simulink model "CIC_manual_test"  (R2016b)
settings: Solver=VariableStepAuto  StartTime=0.0  StopTime=2^16/Fadc  RelTol=1e-3  EnableMultiTasking=on
PreLoadFcn:
  | setup
values from neighbouring files (symbols this model uses):
  Fadc = 614.4e6    (= 614400000)    [setup.m]
libraries: xbsIndex_r4 x26, CryoDetLibCMB x1
settings Model: Creator=Mitch  LastModifiedBy=mdewart
settings OptimizationCC: LifeSpan=inf
settings DebuggingCC: SFUnexpectedBacktrackingDiag=warning  SFNoUnconditionalDefaultTransitionDiag=warning  SFExecutionAtInitializationDiag=none
settings GRTTargetCC: TargetLangStandard=C89/C90 (ANSI)  GeneratePreprocessorConditionals=Disable all
settings ConfigComp: CovMetricSettings=dw  CovHtmlReporting=on  CovSaveCumulativeToWorkspaceVar=on  CovSaveSingleToWorkspaceVar=on  CovExternalEMLEnable=off

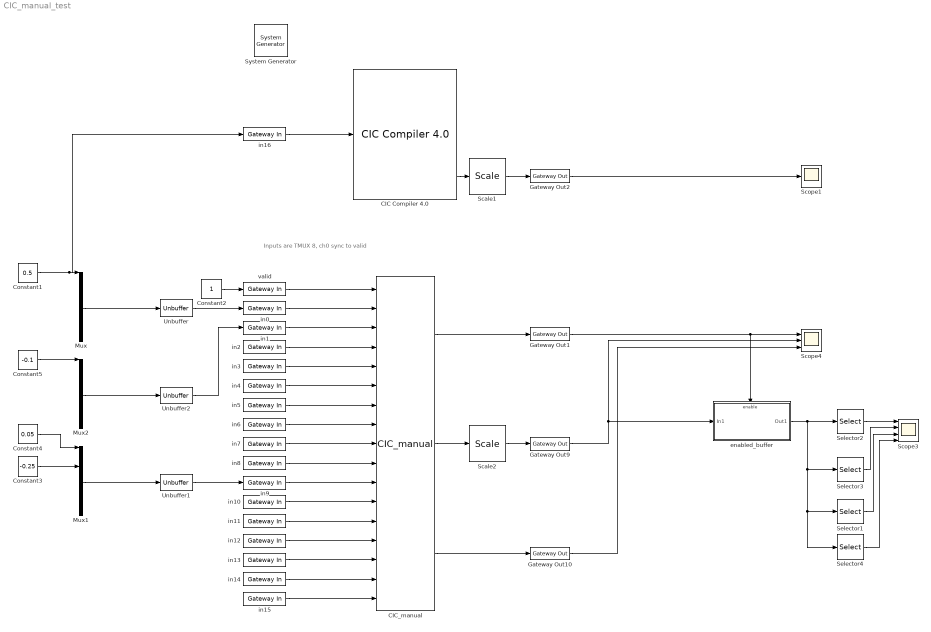
== system CIC_manual_test ==
  note: Inputs are TMUX 8, ch0 sync to valid
  " System Generator" : xbsIndex_r4/ System Generator  Tag=genX  xilinxfamily=kintexu  part=xcku040  speed=-2-e  package=ffva1156  synthesis_tool=Vivado  clock_wrapper=Clock Enables  directory=./netlist  proj_type=Vivado  Synth_file=Vivado Synthesis Defaults  Impl_file=Vivado Implementation Defaults  testbench=off  simulink_period=2/Fadc  sysclk_period=2e9/Fadc  dcm_input_clock_period=10  incr_netlist=off  trim_vbits=Everywhere in SubSystem  dbl_ovrd=According to Block Masks  core_generation=According to Block Masks  run_coregen=off  deprecated_control=off  eval_field=0  block_type=sysgen
  "CIC Compiler 4.0 " : xbsIndex_r4/CIC Compiler 4.0   filter_type=Decimation  number_of_stages=3  differential_delay=1  number_of_channels=1  sample_rate_changes=Fixed  fixed_or_initial_rate=16  minimum_rate=16  maximum_rate=16  ratespecification=Hardware_Oversampling_Rate  sampleperiod=1  hardwareoversamplingrate=1  quantization=Full_Precision  output_data_width=30  use_xtreme_dsp_slice=on  use_streaming_interface=on  has_aclken=off  has_aresetn=off  has_dout_tready=off  trim_axipin_name=on  gui_behaviour=Sysgen_GUI  input_data_width=18  ip_name=CIC Compiler  ip_version=4.0  dsptool_ready=true  wrapper_available=true  port_translation_map={ 'aclken' => 'en', 'aresetn' => 'rst' }  ipcore_xco_need_fpga_part=true  ipcore_verbose=false  block_type=cic_compiler_v4_0
  CIC_manual : CryoDetLibCMB/CIC_manual  n_bit=30  b_pt=15
  Constant1 : Constant  Value=0.5  SampleTime=16/Fadc
  Constant2 : Constant  SampleTime=2/Fadc
  Constant3 : Constant  Value=-0.25  SampleTime=16/Fadc
  Constant4 : Constant  Value=0.05  SampleTime=16/Fadc
  Constant5 : Constant  Value=-0.1  SampleTime=16/Fadc
  Gateway Out{1..2,9..10} (4 alike) : xbsIndex_r4/Gateway Out  inherit_from_input=off  hdl_port=on  rows=1  columns=1  UseAsDAC=off  DACChannel='1'  interface=None  automatic_assignment=on  address_offset=hex2dec('00')  intf_name=''  intf_description=''  timing_constraint=None  locs_specified=off  LOCs={}  io_standard={}  block_type=gatewayout
  Mux : Mux  Inputs=8
  Mux1 : Mux  Inputs=8
  Mux2 : Mux  Inputs=8
  Scale1 : xbsIndex_r4/Scale  scale_factor=-12  dbl_ovrd=off  block_type=scale
  Scale2 : xbsIndex_r4/Scale  scale_factor=-12  dbl_ovrd=off  block_type=scale
  Scope1 : Scope
  Scope3 : Scope  NumInputPorts=4
  Scope4 : Scope  NumInputPorts=3
  Selector1 : Selector  InputPortWidth=128  IndexOptions=Index vector (dialog)  Indices=[9+1]  OutputSizes=1
  Selector2 : Selector  InputPortWidth=128  IndexOptions=Index vector (dialog)  Indices=[0+1]  OutputSizes=1
  Selector3 : Selector  InputPortWidth=128  IndexOptions=Index vector (dialog)  Indices=[1+1]  OutputSizes=1
  Selector4 : Selector  InputPortWidth=128  IndexOptions=Index vector (dialog)  Indices=[41+1]  OutputSizes=1
  Unbuffer : Unbuffer  SampleBasedProcessing=Same as frame based
  Unbuffer1 : Unbuffer  SampleBasedProcessing=Same as frame based
  Unbuffer2 : Unbuffer  SampleBasedProcessing=Same as frame based
  enabled_buffer : Subsystem
  in{0..15} (16 alike) : xbsIndex_r4/Gateway In  gui_display_data_type=Fixed-point  arith_type="Signed  (2's comp)"  n_bits=18  bin_pt=15  preci_type=Single  exp_width=8  frac_width=24  rows=1  columns=1  quantization="Round  (unbiased: +/- Inf)"  overflow=Saturate  period=2/Fadc  UseAsADC=off  ADCChannel='1'  interface=None  automatic_assignment=on  address_offset=hex2dec('00')  intf_name=''  intf_description=''  default_value=0  timing_constraint=None  locs_specified=off  LOCs={}  io_standard={}  inherit_from_input=off  hdl_port=on  dbl_ovrd=off  block_type=gatewayin
  in16 : xbsIndex_r4/Gateway In  gui_display_data_type=Fixed-point  arith_type="Signed  (2's comp)"  n_bits=18  bin_pt=15  preci_type=Single  exp_width=8  frac_width=24  rows=1  columns=1  quantization="Round  (unbiased: +/- Inf)"  overflow=Saturate  period=16/Fadc  UseAsADC=off  ADCChannel='1'  interface=None  automatic_assignment=on  address_offset=hex2dec('00')  intf_name=''  intf_description=''  default_value=0  timing_constraint=None  locs_specified=off  LOCs={}  io_standard={}  inherit_from_input=off  hdl_port=on  dbl_ovrd=off  block_type=gatewayin
  valid : xbsIndex_r4/Gateway In  gui_display_data_type=Boolean  arith_type=Boolean  n_bits=18  bin_pt=15  preci_type=Single  exp_width=8  frac_width=24  rows=1  columns=1  quantization="Round  (unbiased: +/- Inf)"  overflow=Saturate  period=2/Fadc  UseAsADC=off  ADCChannel='1'  interface=None  automatic_assignment=on  address_offset=hex2dec('00')  intf_name=''  intf_description=''  default_value=0  timing_constraint=None  locs_specified=off  LOCs={}  io_standard={}  inherit_from_input=off  hdl_port=on  dbl_ovrd=off  block_type=gatewayin
  wires:
  Constant2/1 -> valid/1
  Constant1/1 -> in16/1, Mux/1
  Mux/1 -> Unbuffer/1
  Unbuffer/1 -> in0/1
  CIC_manual/2 -> Scale2/1
  CIC_manual/3 -> Gateway Out10/1
  CIC_manual/1 -> Gateway Out1/1
  Gateway Out9/1 -> enabled_buffer/1(In1), Scope4/2
  Gateway Out10/1 -> Scope4/3
  Mux1/1 -> Unbuffer1/1
  Constant4/1 -> Mux1/1
  in16/1 -> "CIC Compiler 4.0 "/1
  "CIC Compiler 4.0 "/3 -> Scale1/1
  Gateway Out2/1 -> Scope1/1
  Scale1/1 -> Gateway Out2/1
  Constant3/1 -> Mux1/3
  Selector2/1 -> Scope3/1
  enabled_buffer/1(Out1) -> Selector2/1, Selector3/1, Selector4/1, Selector1/1
  Unbuffer1/1 -> in9/1
  Mux2/1 -> Unbuffer2/1
  Unbuffer2/1 -> in1/1
  Constant5/1 -> Mux2/1
  Selector3/1 -> Scope3/2
  Selector1/1 -> Scope3/3
  Selector4/1 -> Scope3/4
  in7/1 -> CIC_manual/9
  in2/1 -> CIC_manual/4
  in6/1 -> CIC_manual/8
  in15/1 -> CIC_manual/17
  valid/1 -> CIC_manual/1
  in13/1 -> CIC_manual/15
  in11/1 -> CIC_manual/13
  in14/1 -> CIC_manual/16
  in1/1 -> CIC_manual/3
  in8/1 -> CIC_manual/10
  in0/1 -> CIC_manual/2
  in3/1 -> CIC_manual/5
  in9/1 -> CIC_manual/11
  in5/1 -> CIC_manual/7
  in12/1 -> CIC_manual/14
  in4/1 -> CIC_manual/6
  in10/1 -> CIC_manual/12
  Gateway Out1/1 -> enabled_buffer/Enable, Scope4/1
  Scale2/1 -> Gateway Out9/1

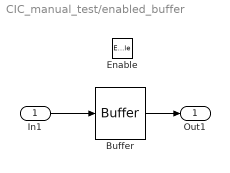
== system CIC_manual_test/enabled_buffer ==
  In1 : Inport
  Enable : EnablePort
  Buffer : Buffer  N=128  TreatMby1Signals=One channel  OutputFrames=off
  Out1 : Outport
  wires:
  Buffer/1 -> Out1/1
  In1/1 -> Buffer/1
